simulink model "ModeloEmBaseNova"  (Simulink 7.1)
settings: Solver=ode45  StartTime=0.0  StopTime=10.0  RelTol=1e-3
undefined symbols (not defined in the file): ANC, BNC, CNC
settings Model: Creator=ALUNO  LastModifiedBy=ALUNO

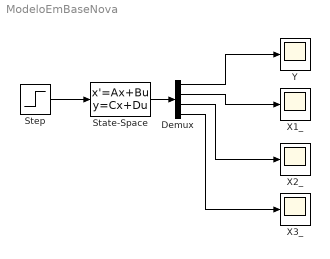
== system ModeloEmBaseNova ==
  Demux : Demux
  State-Space : StateSpace  A=ANC  B=BNC  C=CNC  D=[0;0;0;0]
  Step : Step  SampleTime=0
  X1_ : Scope
  X2_ : Scope
      settings: SaveName=ScopeData2
  X3_ : Scope
      settings: SaveName=ScopeData3
  Y : Scope
  wires:
  Step/1 -> State-Space/1
  State-Space/1 -> Demux/1
  Demux/1 -> Y/1
  Demux/2 -> X1_/1
  Demux/3 -> X2_/1
  Demux/4 -> X3_/1
